simulink model "lane_change"  (R2024a)
settings: Solver=FixedStepAuto  StartTime=0.0  StopTime=10.0  RelTol=1e-3
undefined symbols (not defined in the file): route1_waypoint, route2_waypoint, route3_waypoint, route4_waypoint, route5_waypoint
libraries: CarMaker4SL x9
settings Model: Creator=User  LastModifiedBy=User

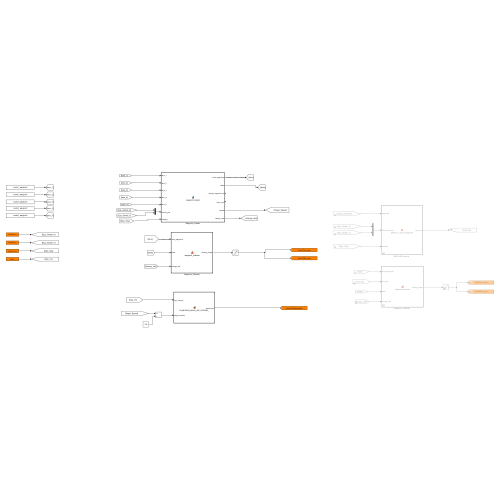
[thumbnail: Simulink's stored preview of the top-level diagram]
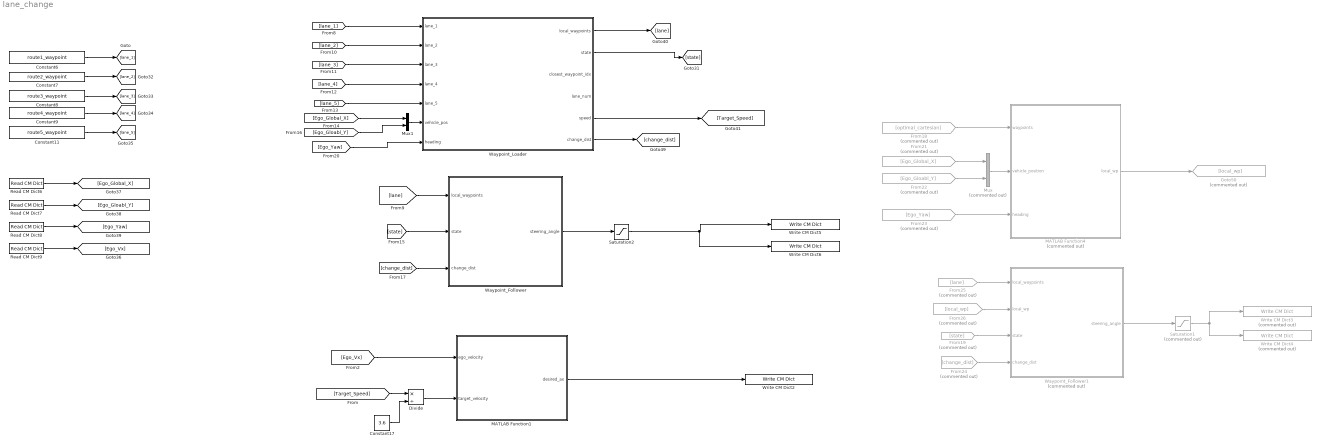
== system lane_change ==
  Constant11 : Constant  Value=route5_waypoint
  Constant17 : Constant  Value=3.6
  Constant6 : Constant  Value=route1_waypoint
  Constant7 : Constant  Value=route2_waypoint
  Constant8 : Constant  Value=route3_waypoint
  Constant9 : Constant  Value=route4_waypoint
  Divide : Product  Inputs=*/
  From18 : From  Commented=on  GotoTag=optimal_cartesian
  From19 : From  Commented=on  GotoTag=state
  From21 : From  Commented=on  GotoTag=Ego_Global_X
  From22 : From  Commented=on  GotoTag=Ego_Gloabl_Y
  From23 : From  Commented=on  GotoTag=Ego_Yaw
  From24 : From  Commented=on  GotoTag=change_dist
  From25 : From  Commented=on  GotoTag=lane
  From26 : From  Commented=on  GotoTag=local_wp
  Goto50 : Goto  Commented=on  GotoTag=local_wp
  MATLAB Function1 : MATLAB Function  TreatAsAtomicUnit=on
  "MATLAB Function4 " : MATLAB Function  Commented=on  TreatAsAtomicUnit=on
  Mux : Mux  Commented=on  Inputs=2
  Mux1 : Mux  Inputs=2
  Read CM Dict6 : CarMaker4SL/Read CM Dict  xname=Car.Fr1.tx  xsync=off  xstime=Inherited
  Read CM Dict7 : CarMaker4SL/Read CM Dict  xname=Car.Fr1.ty  xsync=off  xstime=Inherited
  Read CM Dict8 : CarMaker4SL/Read CM Dict  xname=Car.Fr1.rz  xsync=off  xstime=Inherited
  Read CM Dict9 : CarMaker4SL/Read CM Dict  xname=Car.v  xsync=off  xstime=Inherited
  Saturation1 : Saturate  Commented=on  UpperLimit=2  LowerLimit=-2
  Saturation2 : Saturate  UpperLimit=2  LowerLimit=-2
  Waypoint_Follower : MATLAB Function  TreatAsAtomicUnit=on
  Waypoint_Follower1 : MATLAB Function  Commented=on  TreatAsAtomicUnit=on
  Waypoint_Loader : MATLAB Function  TreatAsAtomicUnit=on
  Write CM Dict2 : CarMaker4SL/Write CM Dict  xname=AccelCtrl.DesiredAx  xsync=off
  Write CM Dict3 : CarMaker4SL/Write CM Dict  Commented=on  xname=Car.CFL.rz_ext  xsync=off
  Write CM Dict4 : CarMaker4SL/Write CM Dict  Commented=on  xname=Car.CFR.rz_ext  xsync=off
  Write CM Dict5 : CarMaker4SL/Write CM Dict  xname=Car.CFL.rz_ext  xsync=off
  Write CM Dict6 : CarMaker4SL/Write CM Dict  xname=Car.CFR.rz_ext  xsync=off
  wires:
  "MATLAB Function4 "/1(local_wp) -> Goto50/1
  From21/1 -> Mux/1
  Mux/1 -> "MATLAB Function4 "/2(vehicle_position)
  From18/1 -> "MATLAB Function4 "/1(waypoints)
  From22/1 -> Mux/2
  From25/1 -> Waypoint_Follower1/1(local_waypoints)
  From23/1 -> "MATLAB Function4 "/3(heading)
  Saturation1/1 -> Write CM Dict3/1, Write CM Dict4/1
  From19/1 -> Waypoint_Follower1/3(state)
  Waypoint_Follower1/1(steering_angle) -> Saturation1/1
  From24/1 -> Waypoint_Follower1/4(change_dist)
  From26/1 -> Waypoint_Follower1/2(local_wp)
  Waypoint_Loader/6(change_dist) -> [change_dist]
  [change_dist] -> Waypoint_Follower/3(change_dist)
  Constant17/1 -> Divide/2
  Divide/1 -> MATLAB Function1/2(target_velocity)
  [Target_Speed] -> Divide/1
  [state] -> Waypoint_Follower/2(state)
  Waypoint_Loader/5(speed) -> [Target_Speed]
  Waypoint_Loader/2(state) -> [state]
  Waypoint_Follower/1(steering_angle) -> Saturation2/1
  [lane] -> Waypoint_Follower/1(local_waypoints)
  [lane_2] -> Waypoint_Loader/2(lane_2)
  Constant9/1 -> [lane_4]
  [Ego_Gloabl_Y] -> Mux1/2
  Constant7/1 -> [lane_2]
  [lane_3] -> Waypoint_Loader/3(lane_3)
  [lane_5] -> Waypoint_Loader/5(lane_5)
  [lane_4] -> Waypoint_Loader/4(lane_4)
  Mux1/1 -> Waypoint_Loader/6(vehicle_pos)
  [Ego_Vx] -> MATLAB Function1/1(ego_velocity)
  Constant8/1 -> [lane_3]
  [lane_1] -> Waypoint_Loader/1(lane_1)
  Saturation2/1 -> Write CM Dict6/1, Write CM Dict5/1
  Read CM Dict8/1 -> [Ego_Yaw]
  Read CM Dict9/1 -> [Ego_Vx]
  Constant6/1 -> [lane_1]
  Read CM Dict6/1 -> [Ego_Global_X]
  Read CM Dict7/1 -> [Ego_Gloabl_Y]
  Waypoint_Loader/1(local_waypoints) -> [lane]
  Constant11/1 -> [lane_5]
  [Ego_Yaw] -> Waypoint_Loader/7(heading)
  [Ego_Global_X] -> Mux1/1
  MATLAB Function1/1(desired_ax) -> Write CM Dict2/1

== matlab function lane_change/MATLAB Function4  ==
  settings: sampleTime=0.1
  data: waypoints input; local_wp output; vehicle_position input; heading input
function local_wp = global_to_local_waypoints(waypoints, vehicle_position, heading)

    waypoints_x = waypoints(:,1);
    waypoints_y = waypoints(:,2);
    num_points = length(waypoints_x);

    local_wp = zeros(num_points, 2);
    x_ego = vehicle_position(1);
    y_ego = vehicle_position(2);
    
    for i = 1:num_points
        dx = waypoints_x(i) - x_ego;
        dy = waypoints_y(i) - y_ego;

        local_x = dx * cos(-heading) - dy * sin(-heading);
        local_y = dx * sin(-heading) + dy * cos(-heading);

        local_wp(i, :) = [local_x, local_y];
    end    
end

== matlab function lane_change/Waypoint_Loader ==
  data: lane_1 input; local_waypoints output; lane_2 input; lane_3 input; lane_4 input; lane_5 input; state output; vehicle_pos input; heading input; closest_waypoint_idx output; lane_num output; speed output; change_dist output
function [local_waypoints, state, closest_waypoint_idx, lane_num, speed, change_dist] = waypoint_loader(lane_1, lane_2, lane_3, lane_4, lane_5, vehicle_pos, heading)
    
    lane_5 = [lane_5; 2.38, -36.18; 3.17, -36.47; 4, -36.6; 4.5, -36.6; 5.0, -36.6; 5.5, -36.6];

    persistent lap_count;
    if isempty(lap_count)
        lap_count = 1;
    end
    persistent entry_5;
    if isempty(entry_5)
        entry_5 = 1;
    end

    lane = lane_2; 
    state = 0;
    lane_num = 0;
    speed = 0;
    change_dist = 0;

    distances = sqrt((lane(:,1) - vehicle_pos(1)).^2 + (lane(:,2) - vehicle_pos(2)).^2);
    [~, closest_waypoint_idx] = min(distances);

    if lap_count == 1
        if closest_waypoint_idx < 18
            lane = lane_2;
            lane_num = 2;
            speed = 50;
        elseif closest_waypoint_idx < 55
            lane = lane_1;
            lane_num = 1;
            speed = 50;
        elseif closest_waypoint_idx < 87
            lane = lane_2;
            lane_num = 2;
            speed = 50;
        elseif closest_waypoint_idx < 125
            lane = lane_1;
            lane_num = 1;
            speed = 50;
        elseif closest_waypoint_idx < 180
            lane = lane_2;
            lane_num = 2;
            state = 0;
            speed = 50;
        elseif closest_waypoint_idx < 190
            lane = lane_1;
            lane_num = 1;
            state = 1;
            speed = 50;
        elseif closest_waypoint_idx < 200
            lane = lane_2;
            lane_num = 2;
            state = 2;
            speed = 50;
        elseif closest_waypoint_idx < 224
            lane = lane_3;
            lane_num = 3;
            state = 3;
            speed = 50;
            lap_count = lap_count + 1;
        else
            lane = lane_2;
            lane_num = 2;
            speed = 50;
        end


    else
        lane = lane_3;
        if closest_waypoint_idx < 9
            lane = lane_3;
            lane_num = 50;
            state = 5;
            speed = 50;
        elseif closest_waypoint_idx < 22
            lane = lane_4;
            lane_num = 80;
            speed = 30;
            entry_5 = entry_5 + 1;
            state = 6;
        elseif entry_5 > 1
            lane = lane_5;
            lane_num = 200;
            state = 7;
            speed = 10;
        else 
            lane = lane_3;
            lane_num = 100; 
            state = 4;
            speed = 50;
        end
    end

    % closest_waypoint 
    distances = sqrt((lane(:,1) - vehicle_pos(1)).^2 + (lane(:,2) - vehicle_pos(2)).^2);
    [~, closest_waypoint_idx] = min(distances);
    start_idx = closest_waypoint_idx;
    
    % lane_change diff dist
    dx_c = lane(closest_waypoint_idx, 1) - vehicle_pos(1);
    dy_c = lane(closest_waypoint_idx, 2) - vehicle_pos(2);
    change_dist = sqrt(dx_c^2 + dy_c^2);

    % 10 waypoint select
    end_idx = min(start_idx + 9, size(lane, 1));
    selected_waypoints = lane(start_idx:end_idx, :);

    % local transform
    local_waypoints = zeros(size(selected_waypoints));
    for i = 1:size(selected_waypoints, 1)
        dx = selected_waypoints(i, 1) - vehicle_pos(1);
        dy = selected_waypoints(i, 2) - vehicle_pos(2);

        local_x = dx * cos(-heading) - dy * sin(-heading);
        local_y = dx * sin(-heading) + dy * cos(-heading);

        local_waypoints(i, :) = [local_x, local_y];
    end
end

% function [local_waypoints, state, closest_waypoint_idx, lane_num] = waypoint_loader(lane_1, lane_2, lane_3, lane_4, lane_5, vehicle_pos, heading)
% 
%     persistent lap_count current_lane_num;
%     if isempty(lap_count)
%         lap_count = 1;
%     end
% 
%     if isempty(current_lane_num)
%         current_lane_num = 2;
%     end
% 
%     lane_list = {lane_1, lane_2, lane_3, lane_4, lane_5};
% 
%     current_lane = lane_list{current_lane_num};
%     distances = sqrt((current_lane(:,1) - vehicle_pos(1)).^2 + (current_lane(:,2) - vehicle_pos(2)).^2);
%     [~, closest_waypoint_idx] = min(distances);
% 
%     if lap_count == 1
%         if  closest_waypoint_idx > 200
%             current_lane_num = 1; 
%         elseif closest_waypoint_idx > 210
%             current_lane_num = 2; 
%         elseif  closest_waypoint_idx > 223
%             current_lane_num = 3;
%             lap_count = lap_count + 1;
%         else 
%             current_lane_num = 2;
%         end
%     else
%         % --- Lap 2 이상 로직 ---
%         if current_lane_num == 3 && closest_waypoint_idx > 10
%             current_lane_num = 4;
%         elseif current_lane_num == 4 && closest_waypoint_idx > 15
%             current_lane_num = 5;
%         end
%     end
% 
%     % 최종 lane 정보
%     lane = lane_list{current_lane_num};
%     lane_num = current_lane_num;
% 
%     % 최신 lane에 대해 closest waypoint 재계산
%     distances = sqrt((lane(:,1) - vehicle_pos(1)).^2 + (lane(:,2) - vehicle_pos(2)).^2);
%     [~, closest_waypoint_idx] = min(distances);
% 
% 
%     start_idx = closest_waypoint_idx;
%     end_idx = min(start_idx + 9, size(lane, 1));
%     selected_waypoints = lane(start_idx:end_idx, :);
% 
%     local_waypoints = zeros(size(selected_waypoints));
%     for i = 1:size(selected_waypoints, 1)
%         dx = selected_waypoints(i, 1) - vehicle_pos(1);
%         dy = selected_waypoints(i, 2) - vehicle_pos(2);
% 
%         local_x = dx * cos(-heading) - dy * sin(-heading);
%         local_y = dx * sin(-heading) + dy * cos(-heading);
% 
%         local_waypoints(i, :) = [local_x, local_y];
%     end
% 
%     state = 0; % 필요에 따라 갱신
% 
% end

== matlab function lane_change/Waypoint_Follower1 ==
  settings: sampleTime=0.1
  data: local_waypoints input; local_wp input; steering_angle output; state input; change_dist input
% local tracking
function steering_angle = waypoint_follower(local_waypoints, local_wp, state, change_dist)

    WHEEL_BASE = 2.9;
    lookahead_dist = 4.5;

    if((state == 1 || state == 2 || state == 3 || state == 4))
        lookahead_dist = 10;
    end

    if(state == 7)
        lookahead_dist = 2.5;
    end

    target_idx = -1;
    final_ld = 0;

    for i = 1:size(local_waypoints, 1)
        dist = norm(local_waypoints(i, :));
        if dist > lookahead_dist && local_waypoints(i, 1) > 0
            target_idx = i;
            final_ld = dist;
            break;
        end
    end

    if target_idx == -1
        steering_angle = 0;
        return;
    end

    target_point = local_waypoints(target_idx, :);
    alpha = atan2(target_point(2), target_point(1));
    alpha = wrapToPi(alpha);

    final_ld = min(max(final_ld, 2.0), 20.0); 

    steering_angle = atan2(2 * WHEEL_BASE * sin(alpha), final_ld);
end

== matlab function lane_change/MATLAB Function1 ==
  settings: sampleTime=0.1
  data: ego_velocity input; desired_ax output; target_velocity input
function desired_ax = longitudinal_speed_pid_controller_(ego_velocity, target_velocity)
    persistent Kp Kd prev_error dt

    % 초기화 (한 번만 실행)
    if isempty(prev_error)
        Kp = 1.0;     % 비례 이득
        Kd = 0.0;     % 미분 이득
        dt = 0.001;    % 제어 주기 (초)
        prev_error = 0;
    end

    % 오차 계산
    error = target_velocity - ego_velocity;
    d_error = (error - prev_error) / dt;

    % PD 제어 계산
    desired_ax = Kp * error + Kd * d_error;

    % 상태 업데이트
    prev_error = error;
end

== matlab function lane_change/Waypoint_Follower ==
  settings: sampleTime=0.1
  data: local_waypoints input; steering_angle output; state input; change_dist input
% local tracking
function steering_angle = waypoint_follower(local_waypoints, state, change_dist)

    WHEEL_BASE = 2.9;
    lookahead_dist = 4.5;
    
    % sigmoid lookahead_dist change
    if(change_dist > 1.8) 
        lookahead_dist = (10 / (1 + exp(-0.4 * change_dist))) + 5;
    end

    % final state -> parking area entry
    if(state == 7)
        lookahead_dist = 2.5;
    end

    target_idx = -1;
    final_ld = 0;

    for i = 1:size(local_waypoints, 1)
        dist = norm(local_waypoints(i, :));
        if dist > lookahead_dist && local_waypoints(i, 1) > 0
            target_idx = i;
            final_ld = dist;
            break;
        end
    end

    if target_idx == -1
        steering_angle = 0;
        return;
    end

    target_point = local_waypoints(target_idx, :);
    alpha = atan2(target_point(2), target_point(1));
    alpha = wrapToPi(alpha);

    final_ld = min(max(final_ld, 2.0), 20.0); 

    steering_angle = atan2(2 * WHEEL_BASE * sin(alpha), final_ld);
end


% % global tracking
% function [steering_angle, start_idx] = pure_pursuit(waypoints, vehicle_position, head)
% 
%     persistent last_target_idx;
%     if isempty(last_target_idx)
%         last_target_idx = 1; % 초기값 설정
%     end
% 
%     WHEEL_BASE = 2.7;
% 
%     waypoints_x = waypoints(:,1);
%     waypoints_y = waypoints(:,2);
%     % num_points = length(waypoints_x);
%     num_points = 300;
% 
%     local_waypoints = zeros(num_points, 2);
%     x_ego = vehicle_position(1);
%     y_ego = vehicle_position(2);
% 
%     for i = 1:num_points
%         dx = waypoints_x(i) - x_ego;
%         dy = waypoints_y(i) - y_ego;
% 
%         local_x = dx * cos(-head) - dy * sin(-head);
%         local_y = dx * sin(-head) + dy * cos(-head);
% 
%         local_waypoints(i, :) = [local_x, local_y];
%     end    
% 
%     lookahead_dist = 5.0;
% 
%     distances_to_waypoints = sqrt((waypoints_x - x_ego).^2 + (waypoints_y - y_ego).^2);
%     [~, closest_idx] = min(distances_to_waypoints);
% 
%     start_idx = max(last_target_idx, closest_idx);
% 
%     target_idx = -1;
%     final_ld = 0;
%     for i = start_idx:num_points
%         dist = norm(local_waypoints(i, :));
%         if dist > lookahead_dist && local_waypoints(i, 1) > 0
%             target_idx = i;
%             final_ld = dist;
%             break;
%         end
%     end
% 
%     if target_idx == -1
%         for i = 1:start_idx-1
%             dist = norm(local_waypoints(i, :));
%             if dist > lookahead_dist && local_waypoints(i, 1) > 0
%                 target_idx = i;
%                 final_ld = dist;
%                 break;
%             end
%         end
%     end
% 
%     if target_idx == -1
%         steering_angle = 0;
%         return;
%     end
% 
%     target_point = local_waypoints(target_idx, :);
%     alpha = atan2(target_point(2), target_point(1));
%     alpha = wrapToPi(alpha);
% 
%     final_ld = min(max(final_ld, 2.0), 20.0);
% 
%     steering_angle = atan2(2 * WHEEL_BASE * sin(alpha), final_ld);
% 
%     last_target_idx = target_idx;
% end
